simulink model "ques9_sys"  (R2020b)
settings: Solver=VariableStepAuto  StartTime=0.0  StopTime=10.0  RelTol=1e-3
values from neighbouring files (symbols this model uses):
  B = 50    [Ques9_code.m]
  J = 15.7*10^-6    (= 1.57e-05)    [Ques9_code.m]
  Kw = 56.23*10^-3    (= 0.05623)    [Ques9_code.m]
  L = 5.05    [Ques9_code.m]
  p = 4    [Ques9_code.m]
  R = 4.98    [Ques9_code.m]
  T1 = 0.1    [Ques9_code.m]
undefined symbols (not defined in the file or in its folder): h2r, Wc
settings Model: Creator=sneha  LastModifiedBy=sneha

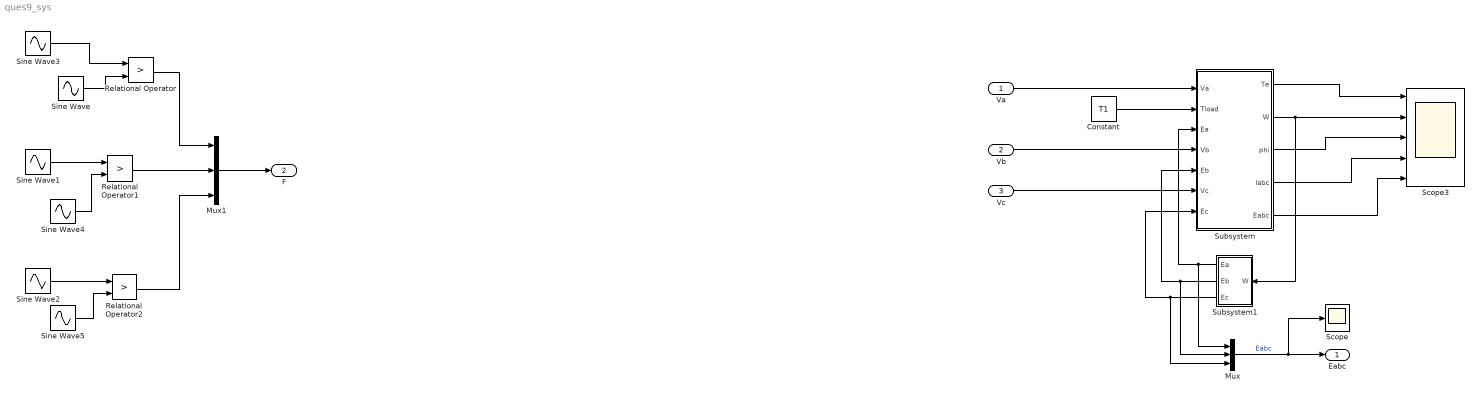
== system ques9_sys ==
  Va : Inport
  Vb : Inport  Port=2
  Vc : Inport  Port=3
  Constant : Constant  Value=T1
  Mux : Mux  Inputs=3
  Mux1 : Mux  Inputs=3
  Relational Operator : RelationalOperator  Operator=>  OutDataTypeStr=boolean  RndMeth=Simplest
  Relational Operator1 : RelationalOperator  Operator=>  OutDataTypeStr=boolean  RndMeth=Simplest
  Relational Operator2 : RelationalOperator  Operator=>  OutDataTypeStr=boolean  RndMeth=Simplest
  Scope : Scope
  Scope3 : Scope  NumInputPorts=5
  Sine Wave : Sin  Frequency=20000*h2r  SampleTime=0
  Sine Wave1 : Sin  Amplitude=0.5  Frequency=50*h2r  Phase=-2*pi/3  SampleTime=0
  Sine Wave2 : Sin  Amplitude=0.5  Frequency=50*h2r  Phase=2*pi/3  SampleTime=0
  Sine Wave3 : Sin  Amplitude=0.5  Frequency=50*h2r  SampleTime=0
  Sine Wave4 : Sin  Frequency=20000*h2r  Phase=-2*pi/3  SampleTime=0
  Sine Wave5 : Sin  Frequency=20000*h2r  Phase=2*pi/3  SampleTime=0
  Subsystem : Subsystem
  Subsystem1 : Subsystem
  Eabc : Outport
  F : Outport  Port=2
  wires:
  Va/1 -> Subsystem/1(Va)
  Constant/1 -> Subsystem/2(Tload)
  Vb/1 -> Subsystem/4(Vb)
  Vc/1 -> Subsystem/6(Vc)
  Subsystem/1(Te) -> Scope3/1
  Subsystem/3(phi) -> Scope3/3
  Subsystem/2(W) -> Subsystem1/1(W), Scope3/2
  Subsystem1/1(Ea) -> Mux/1, Subsystem/3(Ea)
  Subsystem1/2(Eb) -> Mux/2, Subsystem/5(Eb)
  Subsystem1/3(Ec) -> Mux/3, Subsystem/7(Ec)
  Subsystem/4(Iabc) -> Scope3/4
  Subsystem/5(Eabc) -> Scope3/5
  Mux/1 -> Scope/1, Eabc/1  "Eabc"
  Sine Wave2/1 -> Relational Operator2/1
  Sine Wave5/1 -> Relational Operator2/2
  Sine Wave1/1 -> Relational Operator1/1
  Sine Wave4/1 -> Relational Operator1/2
  Sine Wave3/1 -> Relational Operator/1
  Sine Wave/1 -> Relational Operator/2
  Relational Operator/1 -> Mux1/1
  Relational Operator1/1 -> Mux1/2
  Relational Operator2/1 -> Mux1/3
  Mux1/1 -> F/1

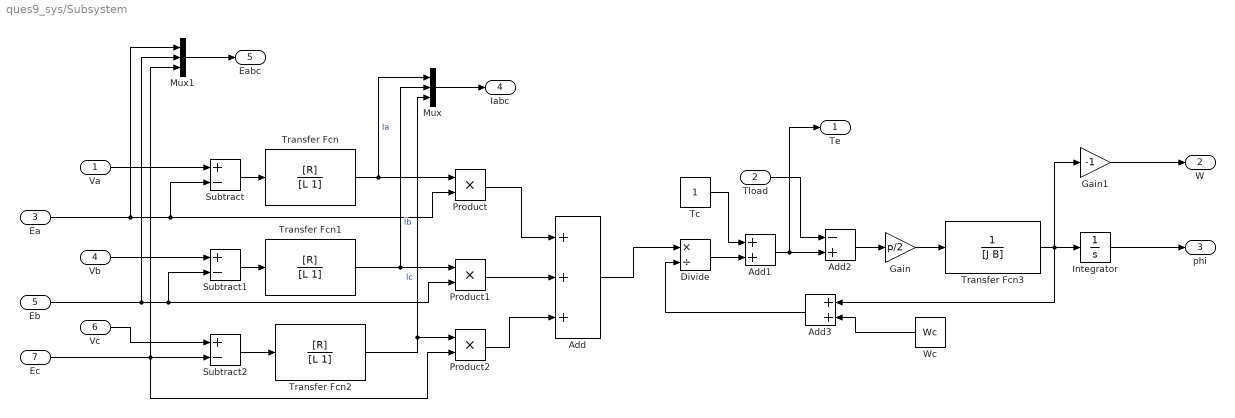
== system ques9_sys/Subsystem ==
  Va : Inport
  Tload : Inport  Port=2
  Ea : Inport  Port=3
  Vb : Inport  Port=4
  Eb : Inport  Port=5
  Vc : Inport  Port=6
  Ec : Inport  Port=7
  Add : Sum  Inputs=+++
  Add1 : Sum
  Add2 : Sum  Inputs=-+
  Add3 : Sum
  Divide : Product  Inputs=*/
  Gain : Gain  Gain=p/2
  Gain1 : Gain  Gain=-1
  Integrator : Integrator
  Mux : Mux  Inputs=3
  Mux1 : Mux  Inputs=3
  Product : Product
  Product1 : Product
  Product2 : Product
  Subtract : Sum  Inputs=+-
  Subtract1 : Sum  Inputs=+-
  Subtract2 : Sum  Inputs=+-
  Tc : Constant
  Transfer Fcn : TransferFcn  Numerator=[R]  Denominator=[L 1]
  Transfer Fcn1 : TransferFcn  Numerator=[R]  Denominator=[L 1]
  Transfer Fcn2 : TransferFcn  Numerator=[R]  Denominator=[L 1]
  Transfer Fcn3 : TransferFcn  Denominator=[J B]
  Wc : Constant  Value=Wc
  Te : Outport
  W : Outport  Port=2
  phi : Outport  Port=3
  Iabc : Outport  Port=4
  Eabc : Outport  Port=5
  wires:
  Transfer Fcn3/1 -> Gain1/1, Add3/1, Integrator/1
  Product2/1 -> Add/3
  Subtract1/1 -> Transfer Fcn1/1
  Subtract/1 -> Transfer Fcn/1
  Add1/1 -> Te/1, Add2/2
  Product1/1 -> Add/2
  Transfer Fcn/1 -> Mux/1, Product/1  "Ia"
  Vb/1 -> Subtract1/1
  Product/1 -> Add/1
  Add/1 -> Divide/1
  Subtract2/1 -> Transfer Fcn2/1
  Add2/1 -> Gain/1
  Gain/1 -> Transfer Fcn3/1
  Transfer Fcn1/1 -> Mux/2, Product1/1  "Ib"
  Ec/1 -> Product2/2, Subtract2/2, Mux1/3
  Divide/1 -> Add1/2
  Transfer Fcn2/1 -> Mux/3, Product2/1  "Ic"
  Tload/1 -> Add2/1
  Tc/1 -> Add1/1
  Wc/1 -> Add3/2
  Add3/1 -> Divide/2
  Integrator/1 -> phi/1
  Gain1/1 -> W/1
  Va/1 -> Subtract/1
  Ea/1 -> Mux1/1, Product/2, Subtract/2
  Vc/1 -> Subtract2/1
  Eb/1 -> Subtract1/2, Product1/2, Mux1/2
  Mux/1 -> Iabc/1
  Mux1/1 -> Eabc/1

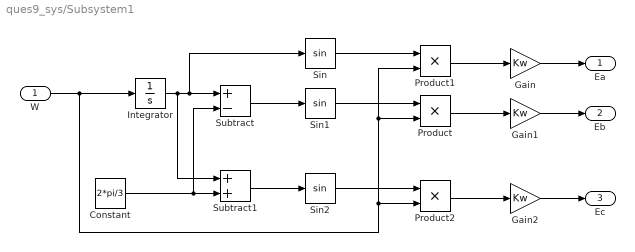
== system ques9_sys/Subsystem1 ==
  W : Inport
  Constant : Constant  Value=2*pi/3
  Gain : Gain  Gain=Kw
  Gain1 : Gain  Gain=Kw
  Gain2 : Gain  Gain=Kw
  Integrator : Integrator
  Product : Product
  Product1 : Product
  Product2 : Product
  Sin : Trigonometry
  Sin1 : Trigonometry
  Sin2 : Trigonometry
  Subtract : Sum  Inputs=+-
  Subtract1 : Sum
  Ea : Outport
  Eb : Outport  Port=2
  Ec : Outport  Port=3
  wires:
  Product2/1 -> Gain2/1
  Sin/1 -> Product1/1
  Constant/1 -> Subtract/2, Subtract1/2
  Subtract1/1 -> Sin2/1
  Product1/1 -> Gain/1
  Subtract/1 -> Sin1/1
  Product/1 -> Gain1/1
  Integrator/1 -> Subtract1/1, Sin/1, Subtract/1
  W/1 -> Integrator/1, Product2/2, Product/2, Product1/2
  Sin1/1 -> Product/1
  Gain1/1 -> Eb/1
  Sin2/1 -> Product2/1
  Gain2/1 -> Ec/1
  Gain/1 -> Ea/1
